simulink model "sk_R3GDL"  (Simulink 8.4)
settings: Solver=ode45  StartTime=0.0  StopTime=10  MaxStep=1e-3  RelTol=1e-3
settings Model: Creator=mortega  LastModifiedBy=etsi  ExtModeTrigMode=oneshot  ExtModeArmWhenConnect=off
settings DataIOCC: LimitDataPoints=off
settings OptimizationCC: BlockReduction=off  BooleanDataType=off  InitFltsAndDblsToZero=on
settings DebuggingCC: SaveWithParameterizedLinksMsg=none  SignalResolutionControl=TryResolveAllWithWarning  SolverPrmCheckMsg=none  MultiTaskDSMMsg=warning  MultiTaskCondExecSysMsg=none
settings HardwareCC: TargetUnknown=on
settings RTWCC: IncludeERTFirstTime=on
settings GRTTargetCC: TargetFcnLib=ansi_tfl_tmw.mat

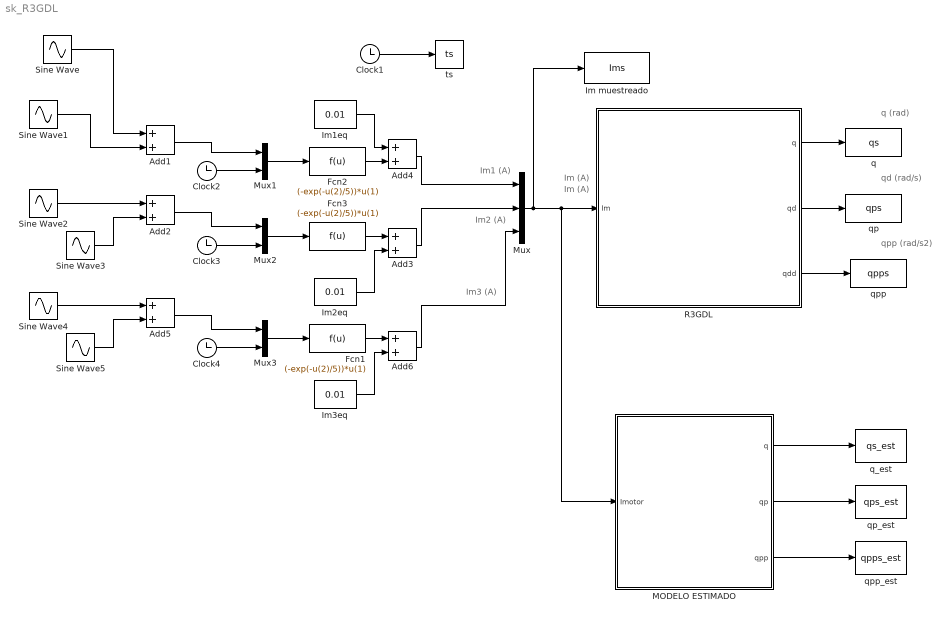
== system sk_R3GDL ==
  note: Im (A)
  note: q (rad)
  note: qd (rad/s)
  note: qpp (rad/s2)
  note: Im (A)
  note: Im1 (A)
  note: Im2 (A)
  note: Im3 (A)
  Add{1..6} (6 alike) : Sum
  Clock{1..4} (4 alike) : Clock
  Fcn1 : Fcn  Expr=(-exp(-u(2)/5))*u(1)
  Fcn2 : Fcn  Expr=(-exp(-u(2)/5))*u(1)
  Fcn3 : Fcn  Expr=(-exp(-u(2)/5))*u(1)
  Im muestreado : ToWorkspace  VariableName=Ims  SampleTime=1e-3
  Im1eq : Constant  Value=0.01
  Im2eq : Constant  Value=0.01
  Im3eq : Constant  Value=0.01
  MODELO ESTIMADO : Subsystem
  Mux : Mux  Inputs=3
  Mux1 : Mux  Inputs=2
  Mux2 : Mux  Inputs=2
  Mux3 : Mux  Inputs=2
  R3GDL : Subsystem  mask(Control y Programación de Robots (4 GIERM)){NGrupo=1, q1_ini=0, q2_ini=0, q3_ini=0, Bl_q1=off, Bl_q2=off, Bl_q3=off, AccionamientoDirecto=off}
      mask prompts: NGrupo "Nº de GRUPO"; q1_ini "q1 inicial  (rad)"; q2_ini "q2 inicial (rad)"; q3_ini "q3_inicial (rad)"; Bl_q1 "Bloqueo q1"; Bl_q2 "Bloqueo q2"; Bl_q3 "Bloqueo q3"; AccionamientoDirecto "Accionamiento directo"
      mask help: Robot de 3 grados de libertad RRR
      mask Display:
      | image(imread('R3GDL_RRR.JPG'));
      | port_label('output', 1, 'q');
      | port_label('output', 2, 'qd');
      | port_label('output', 3, 'qdd');
      | port_label('input', 1, 'Im')
  Sine Wave : Sin  SampleTime=0
  Sine Wave1 : Sin  Amplitude=1.5  Frequency=5  SampleTime=0
  Sine Wave2 : Sin  Frequency=2  SampleTime=0
  Sine Wave3 : Sin  Amplitude=1.5  Frequency=5  SampleTime=0
  Sine Wave4 : Sin  Frequency=2  SampleTime=0
  Sine Wave5 : Sin  Amplitude=1.5  Frequency=5  SampleTime=0
  q : ToWorkspace  VariableName=qs  SampleTime=1e-3
  q_est : ToWorkspace  VariableName=qs_est  SampleTime=1e-3
  qp : ToWorkspace  VariableName=qps  SampleTime=1e-3
  qp_est : ToWorkspace  VariableName=qps_est  SampleTime=1e-3
  qpp : ToWorkspace  VariableName=qpps  SampleTime=1e-3
  qpp_est : ToWorkspace  VariableName=qpps_est  SampleTime=1e-3
  ts : ToWorkspace  VariableName=ts  SampleTime=1e-3
  wires:
  R3GDL/1(q) -> q/1
  R3GDL/2(qd) -> qp/1
  R3GDL/3(qdd) -> qpp/1
  Clock1/1 -> ts/1
  Mux/1 -> MODELO ESTIMADO/1(Imotor), R3GDL/1(Im), Im muestreado/1
  Sine Wave/1 -> Add1/1
  Sine Wave2/1 -> Add2/1
  Sine Wave3/1 -> Add2/2
  Sine Wave1/1 -> Add1/2
  Mux1/1 -> Fcn2/1
  Clock2/1 -> Mux1/2
  Add1/1 -> Mux1/1
  Mux2/1 -> Fcn3/1
  Clock3/1 -> Mux2/2
  Add2/1 -> Mux2/1
  Fcn3/1 -> Add3/1
  Add3/1 -> Mux/2
  Fcn2/1 -> Add4/2
  Add4/1 -> Mux/1
  Im1eq/1 -> Add4/1
  Im2eq/1 -> Add3/2
  Sine Wave5/1 -> Add5/2
  Mux3/1 -> Fcn1/1
  Clock4/1 -> Mux3/2
  Add5/1 -> Mux3/1
  Fcn1/1 -> Add6/1
  Add6/1 -> Mux/3
  Im3eq/1 -> Add6/2
  Sine Wave4/1 -> Add5/1
  MODELO ESTIMADO/1(q) -> q_est/1
  MODELO ESTIMADO/2(qp) -> qp_est/1
  MODELO ESTIMADO/3(qpp) -> qpp_est/1

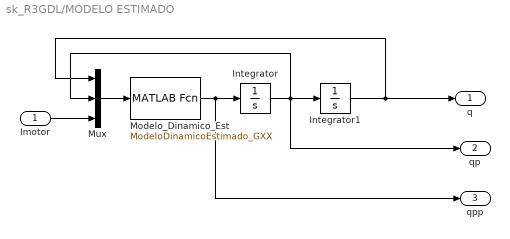
== system sk_R3GDL/MODELO ESTIMADO ==
  Imotor : Inport
  Integrator : Integrator  InitialCondition=[0;0;0]
  Integrator1 : Integrator  InitialCondition=[0;0;0]
  Modelo_Dinamico_Est : MATLABFcn  MATLABFcn=ModeloDinamicoEstimado_GXX  OutputDimensions=3
  Mux : Mux  Inputs=3
  q : Outport
  qp : Outport  Port=2
  qpp : Outport  Port=3
  wires:
  Imotor/1 -> Mux/3
  Integrator1/1 -> Mux/1, q/1
  Integrator/1 -> Mux/2, qp/1, Integrator1/1
  Modelo_Dinamico_Est/1 -> qpp/1, Integrator/1
  Mux/1 -> Modelo_Dinamico_Est/1

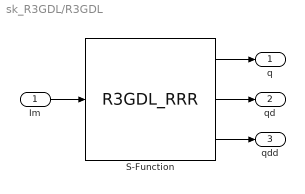
== system sk_R3GDL/R3GDL ==
  Im : Inport
  S-Function : S-Function  FunctionName=R3GDL_RRR  Parameters=[q1_ini; q2_ini; q3_ini]; [Bl_q1; Bl_q2; Bl_q3]; AccionamientoDirecto; NGrupo  EnableBusSupport=off
  q : Outport
  qd : Outport  Port=2
  qdd : Outport  Port=3
  wires:
  Im/1 -> S-Function/1
  S-Function/1 -> q/1
  S-Function/2 -> qd/1
  S-Function/3 -> qdd/1
